simulink model "scara"  (R2023a)
settings: Solver=VariableStepAuto  StartTime=0.0  StopTime=7  MaxStep=1e-3  RelTol=1e-3
model workspace: external: MATLAB File C:\Users\Shantanu Baranwal\Desktop\simscape\scara_DataFile1.m (data not in the file)
undefined symbols (not defined in the file or in its folder): DiscIntNeverNeededParam, K, Lambda, smiData, tau, X, x0, Y, Z
libraries: sm_lib x40, nesl_utility x32, fl_lib x32, slpidlib x6, SignalEditorBlockLib x6, ee_lib x2, simulink x2, spspowerguiLib x1
(part 3 of 3)

== system scara/Subsystem4/Subsystem2/Network Coupler (Flexible Shaft) ==
  note: Uncomment rate transition
      | blocks if one or both networks
      | are running fixed step.
  note: Connect Port 1 to the network
      | with the smaller sample time, or
      | the network running variable step.
  Port 1 Interface : Subsystem  mask(Network Coupler (Flexible Shaft) Port 1 Interface){interfaceModel=an actual shaft compliance, k=0.1, lambda=0.01, samplingType=Variable step at ports 1 and 2, ts=0.001, h1=0.001, h2=0.01, predictionDiscreteToContinuous=off, smoothingContinuousToDiscrete=off, predictionSlowToFast=off, smoothingFastToSlow=off, nSmooth=1, tsSmoothing=0.01, J1=0.01, J2=0.01, tsRecommended=0.0026611, hRecommended=0.00026611, kDerived=250, lambdaDerived=20, tsMax=0.11975, through0=0}
      mask prompts: interfaceModel "physmod:simscape:couplers:SimscapeNetworkCouplersLib:SeparateUsing_MP"; k "physmod:simscape:couplers:SimscapeNetworkCouplersLib:ShaftStiffnessNmrad_MP"; lambda "physmod:simscape:couplers:SimscapeNetworkCouplersLib:ShaftDampingNmrads_MP"; samplingType "physmod:simscape:couplers:SimscapeNetworkCouplersLib:SamplingType_MP"; ts "physmod:simscape:couplers:SimscapeNetworkCouplersLib:SeparatorTimeConstants_MP"; h1 "physmod:simscape:couplers:SimscapeNetworkCouplersLib:Port1NetworkDiscreteSampleTimes_MP"; h2 "physmod:simscape:couplers:SimscapeNetworkCouplersLib:Port2NetworkDiscreteSampleTimes_MP"; predictionDiscreteToContinuous "physmod:simscape:couplers:SimscapeNetworkCouplersLib:UsePredictionWhenConnectingFixedStepToVariableStep_MP"; smoothingContinuousToDiscrete "physmod:simscape:couplers:SimscapeNetworkCouplersLib:UseSmoothingWhenConnectingVariableStepToFixedStep_MP"; predictionSlowToFast "physmod:simscape:couplers:SimscapeNetworkCouplersLib:UsePredictionWhenConnectingSlowToFastSampleTimes_MP"; smoothingFastToSlow "physmod:simscape:couplers:SimscapeNetworkCouplersLib:UseSmoothingWhenConnectingFastToSlowSampleTimes_MP"; nSmooth "physmod:simscape:couplers:SimscapeNetworkCouplersLib:NumberOfSamplesOverWhichToSmooth_MP"; tsSmoothing "physmod:simscape:couplers:SimscapeNetworkCouplersLib:SmoothingTimeConstants_MP"; J1 "physmod:simscape:couplers:SimscapeNetworkCouplersLib:ApproximateInertiaAtPort1kgm2_MP"; J2 "physmod:simscape:couplers:SimscapeNetworkCouplersLib:ApproximateInertiaAtPort2kgm2_MP"; tsRecommended "physmod:simscape:couplers:SimscapeNetworkCouplersLib:RecommendedMaxFilterTimeConstants_MP"; hRecommended "physmod:simscape:couplers:SimscapeNetworkCouplersLib:RecommendedMaxDiscreteSampleTimes_MP"; kDerived "physmod:simscape:couplers:SimscapeNetworkCouplersLib:CalculatedShaftStiffnessNmrad_MP"; lambdaDerived "physmod:simscape:couplers:SimscapeNetworkCouplersLib:CalculatedShaftDampingNmrads_MP"; tsMax "physmod:simscape:couplers:SimscapeNetworkCouplersLib:CalculatedFastestTrackableTimeConstants_MP"; through0 "physmod:simscape:couplers:SimscapeNetworkCouplersLib:InitialTransmittedTorqueNm_MP"
      mask help: physmod:simscape:couplers:SimscapeNetworkCouplersLib:NetworkCouplerFlexibleShaftPort1Interface_MD
      mask init:
      | % Fixed step sample time value check
      | foundation.internal.couplers.checkSampleTimes(gcb,h1,h2);
      | 
      | % Map mask choices to Simscape block parameters  
      | [K,Lambda,tau,~,~,x0,~] = foundation.internal.couplers.mechanical.derivedParamsRotational(...
      |     gcb,ts,h1,h2,through0,k,lambda,J1,J2);
      settings: PortSchema="{\"entries\":[{\"content\":{\"sides\":[{\"content\":{\"connectorIds\":[\"LConn1\"]},\"type\":\"ConnectorPlacement.EquallySpacedRectSide\",\"uuid\":\"a6d4a9fd-b5aa-40dc-ab7e-2b646b9b57bc\"},{\"content\":{\"connectorIds\":[\"Out1\",\"In1\"],\"side\":\"RIGHT\"},\"type\":\"ConnectorPlacement.EquallySpacedRectSide\",\"uuid\":\"31bb6273-5b9b-48d0-a1a2-6fbacb979b97\"},{\"content\":{\"connectorIds\":[],\"side\":\"TOP\"},\"type\":\"ConnectorPlacement.EquallySpacedRectSide\",\"uuid\":\"0f7afab2-4481-486c-9ad0-2b42c5b091a4\"}]},\"type\":\"ConnectorPlacement.EquallySpacedConnector\",\"uuid\":\"a98e47aa-cbfd-441a-b14c-c9ea515c056e\"}],\"packageUris\":[\"http://schema.mathworks.com/mf0/Connector/R2020b\"],\"version\":\"1.0\"}"
      mask Help: web([docroot '/simscape/ref/networkcouplerflexibleshaft.html'])
      mask TypeOptions interfaceModel: physmod:simscape:couplers:SimscapeNetworkCouplersLib:anActualShaftCompliance_PV | physmod:simscape:couplers:SimscapeNetworkCouplersLib:anAddedNumericalCompliance_PV
      mask Callback interfaceModel: foundation.internal.couplers.mechanical.parameterVisibilities(gcb)
      mask TypeOptions samplingType: physmod:simscape:couplers:SimscapeNetworkCouplersLib:VariableStepAtPorts1And2_PV | physmod:simscape:couplers:SimscapeNetworkCouplersLib:VariableStepAtPort1AndFixedStepAtPort2_PV | physmod:simscape:couplers:SimscapeNetworkCouplersLib:FixedStepBothPortsWithCommonSampleTime_PV | physmod:simscape:couplers:SimscapeNetworkCouplersLib:FixedStepBothPortsWithFasterSamplingAtPort1_PV
      mask Callback samplingType: foundation.internal.couplers.mechanical.parameterVisibilities(gcb)
      mask Callback predictionDiscreteToContinuous: foundation.internal.couplers.mechanical.parameterVisibilities(gcb)
      mask Callback smoothingContinuousToDiscrete: foundation.internal.couplers.mechanical.parameterVisibilities(gcb)
      mask Callback predictionSlowToFast: foundation.internal.couplers.mechanical.parameterVisibilities(gcb)
      mask Callback smoothingFastToSlow: foundation.internal.couplers.mechanical.parameterVisibilities(gcb)
      mask DialogControl Main Prompt: Main
      mask DialogControl interfaceModel Prompt: Separate using
      mask DialogControl k Prompt: Shaft stiffness (Nm/rad)
      mask DialogControl lambda Prompt: Shaft damping (Nm/(rad/s))
      mask DialogControl samplingType Prompt: Sampling type
      mask DialogControl ts Prompt: Separator time constant (s)
      mask DialogControl h1 Prompt: Port 1 network discrete sample time (s)
      mask DialogControl h2 Prompt: Port 2 network discrete sample time (s)
      mask DialogControl predictionDiscreteToContinuous Prompt: Use prediction when connecting fixed step to variable step
      mask DialogControl smoothingContinuousToDiscrete Prompt: Use smoothing when connecting variable step to fixed step
      mask DialogControl predictionSlowToFast Prompt: Use prediction when connecting slow to fast sample times
      mask DialogControl smoothingFastToSlow Prompt: Use smoothing when connecting fast to slow sample times
      mask DialogControl nSmooth Prompt: Number of samples over which to smooth
      mask DialogControl tsSmoothing Prompt: Smoothing time constant (s)
      mask DialogControl Analysis Prompt: Analysis
      mask DialogControl connectedNetworkInfo Prompt: Connected network information
      mask DialogControl J1 Prompt: Approximate inertia at port 1 (kg*m^2)
      mask DialogControl J2 Prompt: Approximate inertia at port 2 (kg*m^2)
      mask DialogControl derivedValues Prompt: Derived values
      mask DialogControl tsRecommended Prompt: Recommended max filter time constant (s)
      mask DialogControl hRecommended Prompt: Recommended max discrete sample time (s)
      mask DialogControl kDerived Prompt: Calculated shaft stiffness (Nm/rad)
      mask DialogControl lambdaDerived Prompt: Calculated shaft damping (Nm/(rad/s))
      mask DialogControl tsMax Prompt: Calculated fastest trackable time constant (s)
      mask DialogControl updateRecommendations Prompt: Update
      mask DialogControl updateRecommendations Callback: foundation.internal.couplers.mechanical.analysisRotational(gcb);
      mask DialogControl InitialConditions Prompt: Initial Conditions
      mask DialogControl through0 Prompt: Initial transmitted torque (Nm)
  Port 2 Interface : Subsystem  mask(Network Coupler (Flexible Shaft) Port 2 Interface){}
      mask help: physmod:simscape:couplers:SimscapeNetworkCouplersLib:NetworkCouplerFlexibleShaftPort2Interface_MD
      settings: PortSchema="{\"entries\":[{\"content\":{\"sides\":[{\"content\":{\"connectorIds\":[\"In1\",\"Out1\"]},\"type\":\"ConnectorPlacement.EquallySpacedRectSide\",\"uuid\":\"5a4c1550-e77d-42df-bf3e-b81963920de7\"},{\"content\":{\"connectorIds\":[\"RConn1\"],\"side\":\"RIGHT\"},\"type\":\"ConnectorPlacement.EquallySpacedRectSide\",\"uuid\":\"3fd730f7-5937-4563-a365-595aaae9027b\"},{\"content\":{\"connectorIds\":[],\"side\":\"TOP\"},\"type\":\"ConnectorPlacement.EquallySpacedRectSide\",\"uuid\":\"c16e04e4-26e8-4fd6-98d3-59adbef44c0d\"}]},\"type\":\"ConnectorPlacement.EquallySpacedConnector\",\"uuid\":\"5588d8d0-d459-45fe-a303-1ca6654e99d0\"}],\"packageUris\":[\"http://schema.mathworks.com/mf0/Connector/R2020b\"],\"version\":\"1.0\"}"
      mask Help: web([docroot '/simscape/ref/networkcouplerflexibleshaft.html'])
  Rate transition (fast-to-slow) : RateTransition  Commented=through  Integrity=off
  Rate transition (slow-to-fast) : RateTransition  Commented=through  Integrity=off
  1 : PMIOPort  Side=Left
  2 : PMIOPort  Port=2  Side=Right
  wires:
  Port 1 Interface/1(torque) -> Rate transition (fast-to-slow)/1
  Rate transition (fast-to-slow)/1 -> Port 2 Interface/1(torque)
  Port 2 Interface/1(speed) -> Rate transition (slow-to-fast)/1
  Rate transition (slow-to-fast)/1 -> Port 1 Interface/1(speed)
  connections:
  2/RConn1 -- Port 2 Interface/RConn1
  1/RConn1 -- Port 1 Interface/LConn1

== system scara/Subsystem4/Subsystem3/Network Coupler (Flexible Shaft) ==
  note: Connect Port 1 to the network
      | with the smaller sample time, or
      | the network running variable step.
  note: Uncomment rate transition
      | blocks if one or both networks
      | are running fixed step.
  Port 1 Interface : Subsystem  mask(Network Coupler (Flexible Shaft) Port 1 Interface){interfaceModel=an actual shaft compliance, k=0.1, lambda=0.01, samplingType=Variable step at ports 1 and 2, ts=0.001, h1=0.001, h2=0.01, predictionDiscreteToContinuous=off, smoothingContinuousToDiscrete=off, predictionSlowToFast=off, smoothingFastToSlow=off, nSmooth=1, tsSmoothing=0.01, J1=0.01, J2=0.01, tsRecommended=0.0026611, hRecommended=0.00026611, kDerived=250, lambdaDerived=20, tsMax=0.11975, through0=0}
      mask prompts: interfaceModel "physmod:simscape:couplers:SimscapeNetworkCouplersLib:SeparateUsing_MP"; k "physmod:simscape:couplers:SimscapeNetworkCouplersLib:ShaftStiffnessNmrad_MP"; lambda "physmod:simscape:couplers:SimscapeNetworkCouplersLib:ShaftDampingNmrads_MP"; samplingType "physmod:simscape:couplers:SimscapeNetworkCouplersLib:SamplingType_MP"; ts "physmod:simscape:couplers:SimscapeNetworkCouplersLib:SeparatorTimeConstants_MP"; h1 "physmod:simscape:couplers:SimscapeNetworkCouplersLib:Port1NetworkDiscreteSampleTimes_MP"; h2 "physmod:simscape:couplers:SimscapeNetworkCouplersLib:Port2NetworkDiscreteSampleTimes_MP"; predictionDiscreteToContinuous "physmod:simscape:couplers:SimscapeNetworkCouplersLib:UsePredictionWhenConnectingFixedStepToVariableStep_MP"; smoothingContinuousToDiscrete "physmod:simscape:couplers:SimscapeNetworkCouplersLib:UseSmoothingWhenConnectingVariableStepToFixedStep_MP"; predictionSlowToFast "physmod:simscape:couplers:SimscapeNetworkCouplersLib:UsePredictionWhenConnectingSlowToFastSampleTimes_MP"; smoothingFastToSlow "physmod:simscape:couplers:SimscapeNetworkCouplersLib:UseSmoothingWhenConnectingFastToSlowSampleTimes_MP"; nSmooth "physmod:simscape:couplers:SimscapeNetworkCouplersLib:NumberOfSamplesOverWhichToSmooth_MP"; tsSmoothing "physmod:simscape:couplers:SimscapeNetworkCouplersLib:SmoothingTimeConstants_MP"; J1 "physmod:simscape:couplers:SimscapeNetworkCouplersLib:ApproximateInertiaAtPort1kgm2_MP"; J2 "physmod:simscape:couplers:SimscapeNetworkCouplersLib:ApproximateInertiaAtPort2kgm2_MP"; tsRecommended "physmod:simscape:couplers:SimscapeNetworkCouplersLib:RecommendedMaxFilterTimeConstants_MP"; hRecommended "physmod:simscape:couplers:SimscapeNetworkCouplersLib:RecommendedMaxDiscreteSampleTimes_MP"; kDerived "physmod:simscape:couplers:SimscapeNetworkCouplersLib:CalculatedShaftStiffnessNmrad_MP"; lambdaDerived "physmod:simscape:couplers:SimscapeNetworkCouplersLib:CalculatedShaftDampingNmrads_MP"; tsMax "physmod:simscape:couplers:SimscapeNetworkCouplersLib:CalculatedFastestTrackableTimeConstants_MP"; through0 "physmod:simscape:couplers:SimscapeNetworkCouplersLib:InitialTransmittedTorqueNm_MP"
      mask help: physmod:simscape:couplers:SimscapeNetworkCouplersLib:NetworkCouplerFlexibleShaftPort1Interface_MD
      mask init: same as scara/Subsystem4/Subsystem2/Network Coupler (Flexible Shaft)/Port 1 Interface
      settings: PortSchema="{\"entries\":[{\"content\":{\"sides\":[{\"content\":{\"connectorIds\":[\"LConn1\"]},\"type\":\"ConnectorPlacement.EquallySpacedRectSide\",\"uuid\":\"a6d4a9fd-b5aa-40dc-ab7e-2b646b9b57bc\"},{\"content\":{\"connectorIds\":[\"Out1\",\"In1\"],\"side\":\"RIGHT\"},\"type\":\"ConnectorPlacement.EquallySpacedRectSide\",\"uuid\":\"31bb6273-5b9b-48d0-a1a2-6fbacb979b97\"},{\"content\":{\"connectorIds\":[],\"side\":\"TOP\"},\"type\":\"ConnectorPlacement.EquallySpacedRectSide\",\"uuid\":\"0f7afab2-4481-486c-9ad0-2b42c5b091a4\"}]},\"type\":\"ConnectorPlacement.EquallySpacedConnector\",\"uuid\":\"a98e47aa-cbfd-441a-b14c-c9ea515c056e\"}],\"packageUris\":[\"http://schema.mathworks.com/mf0/Connector/R2020b\"],\"version\":\"1.0\"}"
      mask Help: web([docroot '/simscape/ref/networkcouplerflexibleshaft.html'])
      mask TypeOptions interfaceModel: physmod:simscape:couplers:SimscapeNetworkCouplersLib:anActualShaftCompliance_PV | physmod:simscape:couplers:SimscapeNetworkCouplersLib:anAddedNumericalCompliance_PV
      mask Callback interfaceModel: foundation.internal.couplers.mechanical.parameterVisibilities(gcb)
      mask TypeOptions samplingType: physmod:simscape:couplers:SimscapeNetworkCouplersLib:VariableStepAtPorts1And2_PV | physmod:simscape:couplers:SimscapeNetworkCouplersLib:VariableStepAtPort1AndFixedStepAtPort2_PV | physmod:simscape:couplers:SimscapeNetworkCouplersLib:FixedStepBothPortsWithCommonSampleTime_PV | physmod:simscape:couplers:SimscapeNetworkCouplersLib:FixedStepBothPortsWithFasterSamplingAtPort1_PV
      mask Callback samplingType: foundation.internal.couplers.mechanical.parameterVisibilities(gcb)
      mask Callback predictionDiscreteToContinuous: foundation.internal.couplers.mechanical.parameterVisibilities(gcb)
      mask Callback smoothingContinuousToDiscrete: foundation.internal.couplers.mechanical.parameterVisibilities(gcb)
      mask Callback predictionSlowToFast: foundation.internal.couplers.mechanical.parameterVisibilities(gcb)
      mask Callback smoothingFastToSlow: foundation.internal.couplers.mechanical.parameterVisibilities(gcb)
      mask DialogControl Main Prompt: Main
      mask DialogControl interfaceModel Prompt: Separate using
      mask DialogControl k Prompt: Shaft stiffness (Nm/rad)
      mask DialogControl lambda Prompt: Shaft damping (Nm/(rad/s))
      mask DialogControl samplingType Prompt: Sampling type
      mask DialogControl ts Prompt: Separator time constant (s)
      mask DialogControl h1 Prompt: Port 1 network discrete sample time (s)
      mask DialogControl h2 Prompt: Port 2 network discrete sample time (s)
      mask DialogControl predictionDiscreteToContinuous Prompt: Use prediction when connecting fixed step to variable step
      mask DialogControl smoothingContinuousToDiscrete Prompt: Use smoothing when connecting variable step to fixed step
      mask DialogControl predictionSlowToFast Prompt: Use prediction when connecting slow to fast sample times
      mask DialogControl smoothingFastToSlow Prompt: Use smoothing when connecting fast to slow sample times
      mask DialogControl nSmooth Prompt: Number of samples over which to smooth
      mask DialogControl tsSmoothing Prompt: Smoothing time constant (s)
      mask DialogControl Analysis Prompt: Analysis
      mask DialogControl connectedNetworkInfo Prompt: Connected network information
      mask DialogControl J1 Prompt: Approximate inertia at port 1 (kg*m^2)
      mask DialogControl J2 Prompt: Approximate inertia at port 2 (kg*m^2)
      mask DialogControl derivedValues Prompt: Derived values
      mask DialogControl tsRecommended Prompt: Recommended max filter time constant (s)
      mask DialogControl hRecommended Prompt: Recommended max discrete sample time (s)
      mask DialogControl kDerived Prompt: Calculated shaft stiffness (Nm/rad)
      mask DialogControl lambdaDerived Prompt: Calculated shaft damping (Nm/(rad/s))
      mask DialogControl tsMax Prompt: Calculated fastest trackable time constant (s)
      mask DialogControl updateRecommendations Prompt: Update
      mask DialogControl updateRecommendations Callback: foundation.internal.couplers.mechanical.analysisRotational(gcb);
      mask DialogControl InitialConditions Prompt: Initial Conditions
      mask DialogControl through0 Prompt: Initial transmitted torque (Nm)
  Port 2 Interface : Subsystem  mask(Network Coupler (Flexible Shaft) Port 2 Interface){}
      mask help: physmod:simscape:couplers:SimscapeNetworkCouplersLib:NetworkCouplerFlexibleShaftPort2Interface_MD
      settings: PortSchema="{\"entries\":[{\"content\":{\"sides\":[{\"content\":{\"connectorIds\":[\"In1\",\"Out1\"]},\"type\":\"ConnectorPlacement.EquallySpacedRectSide\",\"uuid\":\"5a4c1550-e77d-42df-bf3e-b81963920de7\"},{\"content\":{\"connectorIds\":[\"RConn1\"],\"side\":\"RIGHT\"},\"type\":\"ConnectorPlacement.EquallySpacedRectSide\",\"uuid\":\"3fd730f7-5937-4563-a365-595aaae9027b\"},{\"content\":{\"connectorIds\":[],\"side\":\"TOP\"},\"type\":\"ConnectorPlacement.EquallySpacedRectSide\",\"uuid\":\"c16e04e4-26e8-4fd6-98d3-59adbef44c0d\"}]},\"type\":\"ConnectorPlacement.EquallySpacedConnector\",\"uuid\":\"5588d8d0-d459-45fe-a303-1ca6654e99d0\"}],\"packageUris\":[\"http://schema.mathworks.com/mf0/Connector/R2020b\"],\"version\":\"1.0\"}"
      mask Help: web([docroot '/simscape/ref/networkcouplerflexibleshaft.html'])
  Rate transition (fast-to-slow) : RateTransition  Commented=through  Integrity=off
  Rate transition (slow-to-fast) : RateTransition  Commented=through  Integrity=off
  1 : PMIOPort  Side=Left
  2 : PMIOPort  Port=2  Side=Right
  wires:
  Rate transition (slow-to-fast)/1 -> Port 1 Interface/1(speed)
  Port 2 Interface/1(speed) -> Rate transition (slow-to-fast)/1
  Rate transition (fast-to-slow)/1 -> Port 2 Interface/1(torque)
  Port 1 Interface/1(torque) -> Rate transition (fast-to-slow)/1
  connections:
  1/RConn1 -- Port 1 Interface/LConn1
  2/RConn1 -- Port 2 Interface/RConn1

== system scara/Subsystem4/Subsystem2/Network Coupler (Flexible Shaft)/Port 1 Interface ==
  speed : Inport
  Ideal Rotational Motion Sensor1 : fl_lib/Mechanical/Mechanical Sensors/Ideal Rotational Motion Sensor  reference=foundation.enum.MeasurementReference.difference  acceleration_port=false  velocity_port=true  position_port=true  wrap_angle=simscape.enum.onoff.off  offset=0 rad
  Interface : Subsystem  Variant=on  VariantControlMode=label  VariantControl=Variant1  LabelModeActiveChoice=Continuous
      settings: PortSchema="{\"entries\":[{\"content\":{\"sides\":[{\"content\":{\"connectorIds\":[\"In1\",\"Out2\"]},\"type\":\"ConnectorPlacement.EquallySpacedRectSide\",\"uuid\":\"aa56821c-7799-44e3-b228-553c5b43a68d\"},{\"content\":{\"connectorIds\":[\"In2\",\"Out1\"],\"side\":\"RIGHT\"},\"type\":\"ConnectorPlacement.EquallySpacedRectSide\",\"uuid\":\"8658dee5-55e2-4f33-bdec-e6600ce27fc1\"},{\"content\":{\"connectorIds\":[],\"side\":\"TOP\"},\"type\":\"ConnectorPlacement.EquallySpacedRectSide\",\"uuid\":\"2effe9c6-8e61-4f0c-a39b-329d9ffc707d\"}]},\"type\":\"ConnectorPlacement.EquallySpacedConnector\",\"uuid\":\"c8fc8444-dfc7-49a5-9550-b957635f7d8f\"}],\"packageUris\":[\"http://schema.mathworks.com/mf0/Connector/R2020b\"],\"version\":\"1.0\"}"
  Mechanical Rotational Reference2 : fl_lib/Mechanical/Rotational Elements/Mechanical Rotational Reference
  Mechanical Rotational Reference3 : fl_lib/Mechanical/Rotational Elements/Mechanical Rotational Reference
  T1 : nesl_utility/Simulink-PS Converter  PhysicalDomain=network_engine_domain  SubClassName=ps_input  LeftPortType=input  RightPortType=output  PseudoPeriodic=off  Frequencies=[]  NoiseDistribution=none  NoiseParameters=[]  Unit=N*m  AffineConversion=off  FilteringAndDerivatives=zero  SimscapeFilterOrder=1  InputFilterTimeConstant=0.001  UdotUserProvided=1
  Tau1 : fl_lib/Mechanical/Mechanical Sources/Ideal Torque Source
  w1 : nesl_utility/PS-Simulink Converter  PhysicalDomain=network_engine_domain  SubClassName=ps_output  LeftPortType=input  RightPortType=output  PseudoPeriodic=off  Frequencies=[]  VectorFormat=1-D array  Unit=rad/s  AffineConversion=off
  1 : PMIOPort  Side=Left
  torque : Outport
  wires:
  Interface/1(through2) -> torque/1
  w1/1 -> Interface/1(across1)
  Interface/2(through1) -> T1/1
  speed/1 -> Interface/2(across2)
  connections:
  T1/RConn1 -- Tau1/RConn1
  Mechanical Rotational Reference3/LConn1 -- Tau1/LConn1
  Ideal Rotational Motion Sensor1/RConn2 -- w1/LConn1
  Mechanical Rotational Reference2/LConn1 -- Ideal Rotational Motion Sensor1/RConn1
  Tau1/RConn2 -- Ideal Rotational Motion Sensor1/LConn1 -- 1/RConn1

== system scara/Subsystem4/Subsystem2/Network Coupler (Flexible Shaft)/Port 2 Interface ==
  torque : Inport
  Ideal Rotational Motion Sensor2 : fl_lib/Mechanical/Mechanical Sensors/Ideal Rotational Motion Sensor  reference=foundation.enum.MeasurementReference.difference  acceleration_port=false  velocity_port=true  position_port=true  wrap_angle=simscape.enum.onoff.off  offset=0 rad
  Mechanical Rotational Reference1 : fl_lib/Mechanical/Rotational Elements/Mechanical Rotational Reference
  Mechanical Rotational Reference4 : fl_lib/Mechanical/Rotational Elements/Mechanical Rotational Reference
  T2 : nesl_utility/Simulink-PS Converter  PhysicalDomain=network_engine_domain  SubClassName=ps_input  LeftPortType=input  RightPortType=output  PseudoPeriodic=off  Frequencies=[]  NoiseDistribution=none  NoiseParameters=[]  Unit=N*m  AffineConversion=off  FilteringAndDerivatives=zero  SimscapeFilterOrder=1  InputFilterTimeConstant=0.001  UdotUserProvided=1
  Tau2 : fl_lib/Mechanical/Mechanical Sources/Ideal Torque Source
  w2 : nesl_utility/PS-Simulink Converter  PhysicalDomain=network_engine_domain  SubClassName=ps_output  LeftPortType=input  RightPortType=output  PseudoPeriodic=off  Frequencies=[]  VectorFormat=1-D array  Unit=rad/s  AffineConversion=off
  2 : PMIOPort  Side=Right
  speed : Outport
  wires:
  w2/1 -> speed/1
  torque/1 -> T2/1
  connections:
  Mechanical Rotational Reference4/LConn1 -- Tau2/LConn1
  Tau2/RConn2 -- 2/RConn1 -- Ideal Rotational Motion Sensor2/LConn1
  Ideal Rotational Motion Sensor2/RConn2 -- w2/LConn1
  Mechanical Rotational Reference1/LConn1 -- Ideal Rotational Motion Sensor2/RConn1
  T2/RConn1 -- Tau2/RConn1

== system scara/Subsystem4/Subsystem3/Network Coupler (Flexible Shaft)/Port 1 Interface ==
  speed : Inport
  Ideal Rotational Motion Sensor1 : fl_lib/Mechanical/Mechanical Sensors/Ideal Rotational Motion Sensor  reference=foundation.enum.MeasurementReference.difference  acceleration_port=false  velocity_port=true  position_port=true  wrap_angle=simscape.enum.onoff.off  offset=0 rad
  Interface : Subsystem  Variant=on  VariantControlMode=label  VariantControl=Variant1  LabelModeActiveChoice=Continuous
      settings: PortSchema="{\"entries\":[{\"content\":{\"sides\":[{\"content\":{\"connectorIds\":[\"In1\",\"Out2\"]},\"type\":\"ConnectorPlacement.EquallySpacedRectSide\",\"uuid\":\"aa56821c-7799-44e3-b228-553c5b43a68d\"},{\"content\":{\"connectorIds\":[\"In2\",\"Out1\"],\"side\":\"RIGHT\"},\"type\":\"ConnectorPlacement.EquallySpacedRectSide\",\"uuid\":\"8658dee5-55e2-4f33-bdec-e6600ce27fc1\"},{\"content\":{\"connectorIds\":[],\"side\":\"TOP\"},\"type\":\"ConnectorPlacement.EquallySpacedRectSide\",\"uuid\":\"2effe9c6-8e61-4f0c-a39b-329d9ffc707d\"}]},\"type\":\"ConnectorPlacement.EquallySpacedConnector\",\"uuid\":\"c8fc8444-dfc7-49a5-9550-b957635f7d8f\"}],\"packageUris\":[\"http://schema.mathworks.com/mf0/Connector/R2020b\"],\"version\":\"1.0\"}"
  Mechanical Rotational Reference2 : fl_lib/Mechanical/Rotational Elements/Mechanical Rotational Reference
  Mechanical Rotational Reference3 : fl_lib/Mechanical/Rotational Elements/Mechanical Rotational Reference
  T1 : nesl_utility/Simulink-PS Converter  PhysicalDomain=network_engine_domain  SubClassName=ps_input  LeftPortType=input  RightPortType=output  PseudoPeriodic=off  Frequencies=[]  NoiseDistribution=none  NoiseParameters=[]  Unit=N*m  AffineConversion=off  FilteringAndDerivatives=zero  SimscapeFilterOrder=1  InputFilterTimeConstant=0.001  UdotUserProvided=1
  Tau1 : fl_lib/Mechanical/Mechanical Sources/Ideal Torque Source
  w1 : nesl_utility/PS-Simulink Converter  PhysicalDomain=network_engine_domain  SubClassName=ps_output  LeftPortType=input  RightPortType=output  PseudoPeriodic=off  Frequencies=[]  VectorFormat=1-D array  Unit=rad/s  AffineConversion=off
  1 : PMIOPort  Side=Left
  torque : Outport
  wires:
  speed/1 -> Interface/2(across2)
  Interface/2(through1) -> T1/1
  w1/1 -> Interface/1(across1)
  Interface/1(through2) -> torque/1
  connections:
  1/RConn1 -- Ideal Rotational Motion Sensor1/LConn1 -- Tau1/RConn2
  Mechanical Rotational Reference2/LConn1 -- Ideal Rotational Motion Sensor1/RConn1
  Ideal Rotational Motion Sensor1/RConn2 -- w1/LConn1
  Mechanical Rotational Reference3/LConn1 -- Tau1/LConn1
  T1/RConn1 -- Tau1/RConn1

== system scara/Subsystem4/Subsystem3/Network Coupler (Flexible Shaft)/Port 2 Interface ==
  torque : Inport
  Ideal Rotational Motion Sensor2 : fl_lib/Mechanical/Mechanical Sensors/Ideal Rotational Motion Sensor  reference=foundation.enum.MeasurementReference.difference  acceleration_port=false  velocity_port=true  position_port=true  wrap_angle=simscape.enum.onoff.off  offset=0 rad
  Mechanical Rotational Reference1 : fl_lib/Mechanical/Rotational Elements/Mechanical Rotational Reference
  Mechanical Rotational Reference4 : fl_lib/Mechanical/Rotational Elements/Mechanical Rotational Reference
  T2 : nesl_utility/Simulink-PS Converter  PhysicalDomain=network_engine_domain  SubClassName=ps_input  LeftPortType=input  RightPortType=output  PseudoPeriodic=off  Frequencies=[]  NoiseDistribution=none  NoiseParameters=[]  Unit=N*m  AffineConversion=off  FilteringAndDerivatives=zero  SimscapeFilterOrder=1  InputFilterTimeConstant=0.001  UdotUserProvided=1
  Tau2 : fl_lib/Mechanical/Mechanical Sources/Ideal Torque Source
  w2 : nesl_utility/PS-Simulink Converter  PhysicalDomain=network_engine_domain  SubClassName=ps_output  LeftPortType=input  RightPortType=output  PseudoPeriodic=off  Frequencies=[]  VectorFormat=1-D array  Unit=rad/s  AffineConversion=off
  2 : PMIOPort  Side=Right
  speed : Outport
  wires:
  torque/1 -> T2/1
  w2/1 -> speed/1
  connections:
  T2/RConn1 -- Tau2/RConn1
  Mechanical Rotational Reference1/LConn1 -- Ideal Rotational Motion Sensor2/RConn1
  Ideal Rotational Motion Sensor2/RConn2 -- w2/LConn1
  Ideal Rotational Motion Sensor2/LConn1 -- 2/RConn1 -- Tau2/RConn2
  Mechanical Rotational Reference4/LConn1 -- Tau2/LConn1

== system scara/Subsystem4/Subsystem2/Network Coupler (Flexible Shaft)/Port 1 Interface/Interface ==
  across1 : Inport
  across2 : Inport  Port=2
  Continuous : Subsystem  VariantControl=Continuous
  Discrete : Subsystem  VariantControl=Discrete
  through2 : Outport
  through1 : Outport  Port=2

== system scara/Subsystem4/Subsystem3/Network Coupler (Flexible Shaft)/Port 1 Interface/Interface ==
  across1 : Inport
  across2 : Inport  Port=2
  Continuous : Subsystem  VariantControl=Continuous
  Discrete : Subsystem  VariantControl=Discrete
  through2 : Outport
  through1 : Outport  Port=2

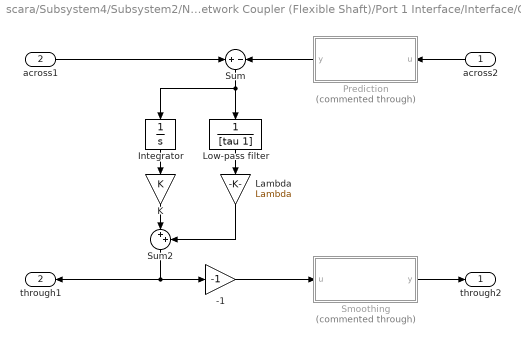
== system scara/Subsystem4/Subsystem2/Network Coupler (Flexible Shaft)/Port 1 Interface/Interface/Continuous ==
  across2 : Inport
  across1 : Inport  Port=2
  -1 : Gain  Gain=-1  SaturateOnIntegerOverflow=on  OutDataTypeStr=Inherit: Same as input  ParamDataTypeStr=Inherit: Same as input
  Integrator : Integrator  InitialCondition=x0
  K : Gain  Gain=K  SaturateOnIntegerOverflow=on  OutDataTypeStr=Inherit: Same as input  ParamDataTypeStr=Inherit: Same as input
  Lambda : Gain  Gain=Lambda  SaturateOnIntegerOverflow=on  OutDataTypeStr=Inherit: Same as input  ParamDataTypeStr=Inherit: Same as input
  Low-pass filter : TransferFcn  Numerator=1  Denominator=[tau 1]
  Prediction : Subsystem  Commented=through  mask(Prediction (discrete->continuous)){h2=h2}
      mask prompts: h2 "physmod:simscape:couplers:SimscapeNetworkCouplersLib:PortUDiscreteSampleTimes_MP"
      mask help: physmod:simscape:couplers:SimscapeNetworkCouplersLib:Predictiondiscretecontinuous_MD
      mask DialogControl h2 Prompt: Port u discrete sample time (s)
  Smoothing : Subsystem  Commented=through  mask(Smoothing (continuous->discrete)){tsSmoothing=tsSmoothing, smoothing0=-through0}
      mask prompts: tsSmoothing "physmod:simscape:couplers:SimscapeNetworkCouplersLib:SmoothingTimeConstants_MP"; smoothing0 "physmod:simscape:couplers:SimscapeNetworkCouplersLib:InitialOutput_MP"
      mask help: physmod:simscape:couplers:SimscapeNetworkCouplersLib:Smoothingcontinuousdiscrete_MD
      mask DialogControl tsSmoothing Prompt: Smoothing time constant (s)
      mask DialogControl smoothing0 Prompt: Initial output
  Sum : Sum  Inputs=+-  InputSameDT=on  SaturateOnIntegerOverflow=on  OutDataTypeStr=Inherit: Same as first input
  Sum2 : Sum  Inputs=|++
  through2 : Outport
  through1 : Outport  Port=2
  wires:
  -1/1 -> Smoothing/1(u)
  Smoothing/1(y) -> through2/1
  Prediction/1(y) -> Sum/2
  Lambda/1 -> Sum2/2
  across1/1 -> Sum/1
  Sum/1 -> Low-pass filter/1, Integrator/1
  Integrator/1 -> K/1
  Low-pass filter/1 -> Lambda/1
  across2/1 -> Prediction/1(u)
  Sum2/1 -> -1/1, through1/1
  K/1 -> Sum2/1

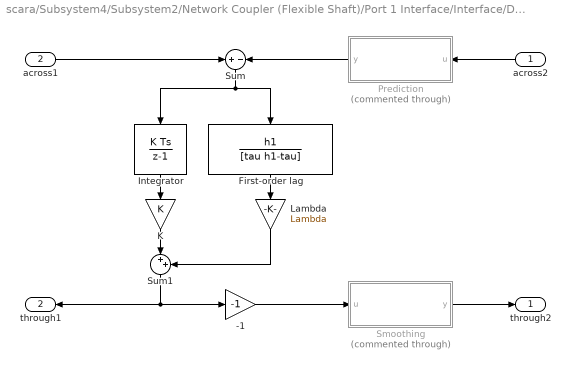
== system scara/Subsystem4/Subsystem2/Network Coupler (Flexible Shaft)/Port 1 Interface/Interface/Discrete ==
  across2 : Inport
  across1 : Inport  Port=2
  -1 : Gain  Gain=-1  SaturateOnIntegerOverflow=on  OutDataTypeStr=Inherit: Same as input  ParamDataTypeStr=Inherit: Same as input
  First-order lag : DiscreteTransferFcn  Numerator=h1  Denominator=[tau h1-tau]  SampleTime=h1
  Integrator : DiscreteIntegrator  InitialCondition=x0  SampleTime=h1  ICPrevOutput=DiscIntNeverNeededParam  ICPrevScaledInput=DiscIntNeverNeededParam
  K : Gain  Gain=K  SaturateOnIntegerOverflow=on  OutDataTypeStr=Inherit: Same as input  ParamDataTypeStr=Inherit: Same as input
  Lambda : Gain  Gain=Lambda  SaturateOnIntegerOverflow=on  OutDataTypeStr=Inherit: Same as input  ParamDataTypeStr=Inherit: Same as input
  Prediction : Subsystem  Commented=through  mask(Prediction (slow->fast)){h2=h2, h1=h1}
      mask prompts: h2 "physmod:simscape:couplers:SimscapeNetworkCouplersLib:PortUDiscreteSampleTimes_MP"; h1 "physmod:simscape:couplers:SimscapeNetworkCouplersLib:PortYDiscreteSampleTimes_MP"
      mask help: physmod:simscape:couplers:SimscapeNetworkCouplersLib:Predictionslowfast_MD
      mask DialogControl h2 Prompt: Port u discrete sample time (s)
      mask DialogControl h1 Prompt: Port y discrete sample time (s)
  Smoothing : Subsystem  Commented=through  mask(Smoothing (fast->slow)){nSmooth=nSmooth, h1=h1, smoothing0=-through0}
      mask prompts: nSmooth "physmod:simscape:couplers:SimscapeNetworkCouplersLib:NumberOfSamplesOverWhichToSmooth_MP"; h1 "physmod:simscape:couplers:SimscapeNetworkCouplersLib:PortUDiscreteSampleTimes_MP"; smoothing0 "physmod:simscape:couplers:SimscapeNetworkCouplersLib:InitialOutput_MP"
      mask help: physmod:simscape:couplers:SimscapeNetworkCouplersLib:Smoothingfastslow_MD
      mask DialogControl nSmooth Prompt: Number of samples over which to smooth
      mask DialogControl h1 Prompt: Port u discrete sample time (s)
      mask DialogControl smoothing0 Prompt: Initial output
  Sum : Sum  Inputs=+-  InputSameDT=on  SaturateOnIntegerOverflow=on  OutDataTypeStr=Inherit: Same as first input
  Sum1 : Sum  Inputs=|++
  through2 : Outport
  through1 : Outport  Port=2
  wires:
  -1/1 -> Smoothing/1(u)
  Smoothing/1(y) -> through2/1
  Prediction/1(y) -> Sum/2
  Lambda/1 -> Sum1/2
  Sum1/1 -> -1/1, through1/1
  across2/1 -> Prediction/1(u)
  Sum/1 -> First-order lag/1, Integrator/1
  across1/1 -> Sum/1
  K/1 -> Sum1/1
  Integrator/1 -> K/1
  First-order lag/1 -> Lambda/1

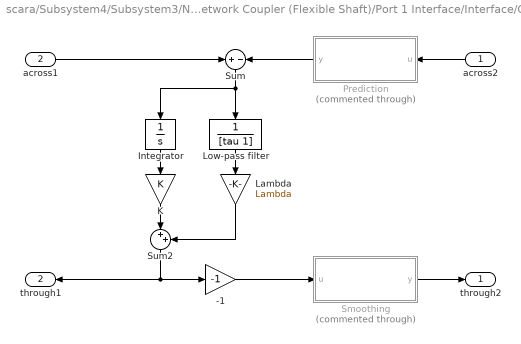
== system scara/Subsystem4/Subsystem3/Network Coupler (Flexible Shaft)/Port 1 Interface/Interface/Continuous ==
  across2 : Inport
  across1 : Inport  Port=2
  -1 : Gain  Gain=-1  SaturateOnIntegerOverflow=on  OutDataTypeStr=Inherit: Same as input  ParamDataTypeStr=Inherit: Same as input
  Integrator : Integrator  InitialCondition=x0
  K : Gain  Gain=K  SaturateOnIntegerOverflow=on  OutDataTypeStr=Inherit: Same as input  ParamDataTypeStr=Inherit: Same as input
  Lambda : Gain  Gain=Lambda  SaturateOnIntegerOverflow=on  OutDataTypeStr=Inherit: Same as input  ParamDataTypeStr=Inherit: Same as input
  Low-pass filter : TransferFcn  Numerator=1  Denominator=[tau 1]
  Prediction : Subsystem  Commented=through  mask(Prediction (discrete->continuous)){h2=h2}
      mask prompts: h2 "physmod:simscape:couplers:SimscapeNetworkCouplersLib:PortUDiscreteSampleTimes_MP"
      mask help: physmod:simscape:couplers:SimscapeNetworkCouplersLib:Predictiondiscretecontinuous_MD
      mask DialogControl h2 Prompt: Port u discrete sample time (s)
  Smoothing : Subsystem  Commented=through  mask(Smoothing (continuous->discrete)){tsSmoothing=tsSmoothing, smoothing0=-through0}
      mask prompts: tsSmoothing "physmod:simscape:couplers:SimscapeNetworkCouplersLib:SmoothingTimeConstants_MP"; smoothing0 "physmod:simscape:couplers:SimscapeNetworkCouplersLib:InitialOutput_MP"
      mask help: physmod:simscape:couplers:SimscapeNetworkCouplersLib:Smoothingcontinuousdiscrete_MD
      mask DialogControl tsSmoothing Prompt: Smoothing time constant (s)
      mask DialogControl smoothing0 Prompt: Initial output
  Sum : Sum  Inputs=+-  InputSameDT=on  SaturateOnIntegerOverflow=on  OutDataTypeStr=Inherit: Same as first input
  Sum2 : Sum  Inputs=|++
  through2 : Outport
  through1 : Outport  Port=2
  wires:
  K/1 -> Sum2/1
  Sum2/1 -> through1/1, -1/1
  across2/1 -> Prediction/1(u)
  Low-pass filter/1 -> Lambda/1
  Integrator/1 -> K/1
  Sum/1 -> Integrator/1, Low-pass filter/1
  across1/1 -> Sum/1
  Lambda/1 -> Sum2/2
  Prediction/1(y) -> Sum/2
  Smoothing/1(y) -> through2/1
  -1/1 -> Smoothing/1(u)

== system scara/Subsystem4/Subsystem3/Network Coupler (Flexible Shaft)/Port 1 Interface/Interface/Discrete ==
  across2 : Inport
  across1 : Inport  Port=2
  -1 : Gain  Gain=-1  SaturateOnIntegerOverflow=on  OutDataTypeStr=Inherit: Same as input  ParamDataTypeStr=Inherit: Same as input
  First-order lag : DiscreteTransferFcn  Numerator=h1  Denominator=[tau h1-tau]  SampleTime=h1
  Integrator : DiscreteIntegrator  InitialCondition=x0  SampleTime=h1  ICPrevOutput=DiscIntNeverNeededParam  ICPrevScaledInput=DiscIntNeverNeededParam
  K : Gain  Gain=K  SaturateOnIntegerOverflow=on  OutDataTypeStr=Inherit: Same as input  ParamDataTypeStr=Inherit: Same as input
  Lambda : Gain  Gain=Lambda  SaturateOnIntegerOverflow=on  OutDataTypeStr=Inherit: Same as input  ParamDataTypeStr=Inherit: Same as input
  Prediction : Subsystem  Commented=through  mask(Prediction (slow->fast)){h2=h2, h1=h1}
      mask prompts: h2 "physmod:simscape:couplers:SimscapeNetworkCouplersLib:PortUDiscreteSampleTimes_MP"; h1 "physmod:simscape:couplers:SimscapeNetworkCouplersLib:PortYDiscreteSampleTimes_MP"
      mask help: physmod:simscape:couplers:SimscapeNetworkCouplersLib:Predictionslowfast_MD
      mask DialogControl h2 Prompt: Port u discrete sample time (s)
      mask DialogControl h1 Prompt: Port y discrete sample time (s)
  Smoothing : Subsystem  Commented=through  mask(Smoothing (fast->slow)){nSmooth=nSmooth, h1=h1, smoothing0=-through0}
      mask prompts: nSmooth "physmod:simscape:couplers:SimscapeNetworkCouplersLib:NumberOfSamplesOverWhichToSmooth_MP"; h1 "physmod:simscape:couplers:SimscapeNetworkCouplersLib:PortUDiscreteSampleTimes_MP"; smoothing0 "physmod:simscape:couplers:SimscapeNetworkCouplersLib:InitialOutput_MP"
      mask help: physmod:simscape:couplers:SimscapeNetworkCouplersLib:Smoothingfastslow_MD
      mask DialogControl nSmooth Prompt: Number of samples over which to smooth
      mask DialogControl h1 Prompt: Port u discrete sample time (s)
      mask DialogControl smoothing0 Prompt: Initial output
  Sum : Sum  Inputs=+-  InputSameDT=on  SaturateOnIntegerOverflow=on  OutDataTypeStr=Inherit: Same as first input
  Sum1 : Sum  Inputs=|++
  through2 : Outport
  through1 : Outport  Port=2
  wires:
  First-order lag/1 -> Lambda/1
  Integrator/1 -> K/1
  K/1 -> Sum1/1
  across1/1 -> Sum/1
  Sum/1 -> Integrator/1, First-order lag/1
  across2/1 -> Prediction/1(u)
  Sum1/1 -> through1/1, -1/1
  Lambda/1 -> Sum1/2
  Prediction/1(y) -> Sum/2
  Smoothing/1(y) -> through2/1
  -1/1 -> Smoothing/1(u)

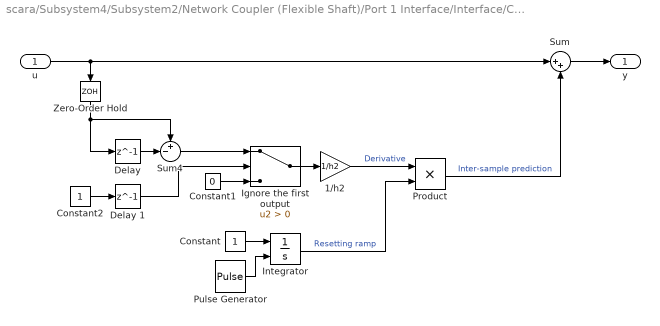
== system scara/Subsystem4/Subsystem2/Network Coupler (Flexible Shaft)/Port 1 Interface/Interface/Continuous/Prediction ==
  u : Inport
  1/h2 : Gain  Gain=1/h2
  Constant : Constant  SampleTime=h2
  Constant1 : Constant  Value=0  SampleTime=h2
  Constant2 : Constant  SampleTime=h2
  "Delay " : Delay  DelayLength=1  SampleTime=h2
  Delay 1 : Delay  DelayLength=1  SampleTime=h2
  Ignore the first output : Switch  Criteria=u2 > Threshold  SaturateOnIntegerOverflow=off  InputSameDT=off
  Integrator : Integrator  ExternalReset=either  LimitOutput=on  UpperSaturationLimit=1  LowerSaturationLimit=0
  Product : Product
  Pulse Generator : DiscretePulseGenerator  SampleTime=h2
  Sum : Sum  Inputs=|++
  Sum4 : Sum  Inputs=+-|
  Zero-Order Hold : ZeroOrderHold  SampleTime=h2
  y : Outport
  wires:
  Constant2/1 -> Delay 1/1
  Delay 1/1 -> Ignore the first output/2
  Constant1/1 -> Ignore the first output/3
  Sum4/1 -> Ignore the first output/1
  Ignore the first output/1 -> 1/h2/1
  Pulse Generator/1 -> Integrator/2
  Constant/1 -> Integrator/1
  Integrator/1 -> Product/2  "Resetting ramp"
  Sum/1 -> y/1
  1/h2/1 -> Product/1  "Derivative"
  "Delay "/1 -> Sum4/2
  u/1 -> Zero-Order Hold/1, Sum/1
  Zero-Order Hold/1 -> "Delay "/1, Sum4/1
  Product/1 -> Sum/2  "Inter-sample prediction"

== system scara/Subsystem4/Subsystem2/Network Coupler (Flexible Shaft)/Port 1 Interface/Interface/Continuous/Smoothing ==
  u : Inport
  Gain : Gain  Gain=1/tsSmoothing
  Integrator : Integrator  InitialCondition=smoothing0
  Sum : Sum  Inputs=|+-
  y : Outport
  wires:
  Sum/1 -> Gain/1
  Gain/1 -> Integrator/1
  Integrator/1 -> y/1, Sum/2
  u/1 -> Sum/1

== system scara/Subsystem4/Subsystem2/Network Coupler (Flexible Shaft)/Port 1 Interface/Interface/Discrete/Prediction ==
  u : Inport
  Constant : Constant  Value=0  SampleTime=h1
  Constant2 : Constant  Value=h1  SampleTime=h1
  "Delay " : Delay  DelayLength=1  SampleTime=h1
  Product : Product
  Resettable Delay : Delay  DelayLength=1  InitialConditionSource=Input port  ExternalReset=Rising  SampleTime=h1
      settings: InputPortMap=u0,r5,p4
  Sum : Sum  Inputs=|++
  Sum1 : Sum  Inputs=|++
  Sum4 : Sum  Inputs=+-|
  Update derivative estimate : Subsystem  TreatAsAtomicUnit=on
  y : Outport
  wires:
  Update derivative estimate/1(Out1) -> Product/1
  u/1 -> Sum/1, Sum4/1, Update derivative estimate/1(u), "Delay "/1
  "Delay "/1 -> Sum4/2
  Sum4/1 -> Update derivative estimate/Trigger, Resettable Delay/2  "Trigger when input changes"
  Sum1/1 -> Resettable Delay/1
  Resettable Delay/1 -> Product/2, Sum1/2
  Constant2/1 -> Sum1/1
  Constant/1 -> Resettable Delay/3
  Sum/1 -> y/1
  Product/1 -> Sum/2

== system scara/Subsystem4/Subsystem2/Network Coupler (Flexible Shaft)/Port 1 Interface/Interface/Discrete/Smoothing ==
  u : Inport
  Gain : Gain  Gain=1/nSmooth
  Sum of Elements : Sum  Inputs=+
  Tapped Delay : simulink/Discrete/Tapped Delay  vinit=smoothing0  samptime=h1  NumDelays=nSmooth  DelayOrder=Oldest  includeCurrent=off
  y : Outport
  wires:
  u/1 -> Tapped Delay/1
  Tapped Delay/1 -> Sum of Elements/1
  Sum of Elements/1 -> Gain/1
  Gain/1 -> y/1

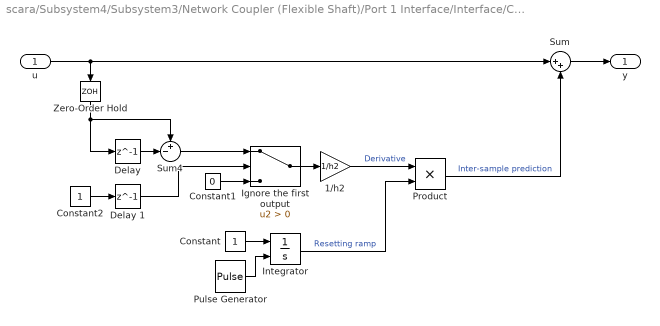
== system scara/Subsystem4/Subsystem3/Network Coupler (Flexible Shaft)/Port 1 Interface/Interface/Continuous/Prediction ==
  u : Inport
  1/h2 : Gain  Gain=1/h2
  Constant : Constant  SampleTime=h2
  Constant1 : Constant  Value=0  SampleTime=h2
  Constant2 : Constant  SampleTime=h2
  "Delay " : Delay  DelayLength=1  SampleTime=h2
  Delay 1 : Delay  DelayLength=1  SampleTime=h2
  Ignore the first output : Switch  Criteria=u2 > Threshold  SaturateOnIntegerOverflow=off  InputSameDT=off
  Integrator : Integrator  ExternalReset=either  LimitOutput=on  UpperSaturationLimit=1  LowerSaturationLimit=0
  Product : Product
  Pulse Generator : DiscretePulseGenerator  SampleTime=h2
  Sum : Sum  Inputs=|++
  Sum4 : Sum  Inputs=+-|
  Zero-Order Hold : ZeroOrderHold  SampleTime=h2
  y : Outport
  wires:
  Product/1 -> Sum/2  "Inter-sample prediction"
  Zero-Order Hold/1 -> Sum4/1, "Delay "/1
  u/1 -> Sum/1, Zero-Order Hold/1
  "Delay "/1 -> Sum4/2
  1/h2/1 -> Product/1  "Derivative"
  Sum/1 -> y/1
  Integrator/1 -> Product/2  "Resetting ramp"
  Constant/1 -> Integrator/1
  Pulse Generator/1 -> Integrator/2
  Ignore the first output/1 -> 1/h2/1
  Sum4/1 -> Ignore the first output/1
  Constant1/1 -> Ignore the first output/3
  Delay 1/1 -> Ignore the first output/2
  Constant2/1 -> Delay 1/1

== system scara/Subsystem4/Subsystem3/Network Coupler (Flexible Shaft)/Port 1 Interface/Interface/Continuous/Smoothing ==
  u : Inport
  Gain : Gain  Gain=1/tsSmoothing
  Integrator : Integrator  InitialCondition=smoothing0
  Sum : Sum  Inputs=|+-
  y : Outport
  wires:
  u/1 -> Sum/1
  Integrator/1 -> Sum/2, y/1
  Gain/1 -> Integrator/1
  Sum/1 -> Gain/1

== system scara/Subsystem4/Subsystem3/Network Coupler (Flexible Shaft)/Port 1 Interface/Interface/Discrete/Prediction ==
  u : Inport
  Constant : Constant  Value=0  SampleTime=h1
  Constant2 : Constant  Value=h1  SampleTime=h1
  "Delay " : Delay  DelayLength=1  SampleTime=h1
  Product : Product
  Resettable Delay : Delay  DelayLength=1  InitialConditionSource=Input port  ExternalReset=Rising  SampleTime=h1
      settings: InputPortMap=u0,r5,p4
  Sum : Sum  Inputs=|++
  Sum1 : Sum  Inputs=|++
  Sum4 : Sum  Inputs=+-|
  Update derivative estimate : Subsystem  TreatAsAtomicUnit=on
  y : Outport
  wires:
  Product/1 -> Sum/2
  Sum/1 -> y/1
  Constant/1 -> Resettable Delay/3
  Constant2/1 -> Sum1/1
  Resettable Delay/1 -> Sum1/2, Product/2
  Sum1/1 -> Resettable Delay/1
  Sum4/1 -> Resettable Delay/2, Update derivative estimate/Trigger  "Trigger when input changes"
  "Delay "/1 -> Sum4/2
  u/1 -> "Delay "/1, Update derivative estimate/1(u), Sum4/1, Sum/1
  Update derivative estimate/1(Out1) -> Product/1

== system scara/Subsystem4/Subsystem3/Network Coupler (Flexible Shaft)/Port 1 Interface/Interface/Discrete/Smoothing ==
  u : Inport
  Gain : Gain  Gain=1/nSmooth
  Sum of Elements : Sum  Inputs=+
  Tapped Delay : simulink/Discrete/Tapped Delay  vinit=smoothing0  samptime=h1  NumDelays=nSmooth  DelayOrder=Oldest  includeCurrent=off
  y : Outport
  wires:
  Gain/1 -> y/1
  Sum of Elements/1 -> Gain/1
  Tapped Delay/1 -> Sum of Elements/1
  u/1 -> Tapped Delay/1

== system scara/Subsystem4/Subsystem2/Network Coupler (Flexible Shaft)/Port 1 Interface/Interface/Discrete/Prediction/Update derivative estimate ==
  u : Inport
  Trigger : TriggerPort  VariantControl=(inherit)
  1/h2 : Gain  Gain=1/h2
  Constant : Constant  Value=0  SampleTime=-1
  Constant1 : Constant  SampleTime=-1
  Sum : Sum  Inputs=|-+
  Switch : Switch  Criteria=u2 > Threshold  SaturateOnIntegerOverflow=off  InputSameDT=off
  Unit Delay : UnitDelay  SampleTime=-1  HasFrameUpgradeWarning=on
  Wait one sample : UnitDelay  SampleTime=-1  HasFrameUpgradeWarning=on
  Out1 : Outport
  wires:
  Constant1/1 -> Wait one sample/1
  Wait one sample/1 -> Switch/2
  Constant/1 -> Switch/3
  Sum/1 -> Switch/1
  Switch/1 -> 1/h2/1
  1/h2/1 -> Out1/1
  u/1 -> Sum/2, Unit Delay/1
  Unit Delay/1 -> Sum/1

== system scara/Subsystem4/Subsystem3/Network Coupler (Flexible Shaft)/Port 1 Interface/Interface/Discrete/Prediction/Update derivative estimate ==
  u : Inport
  Trigger : TriggerPort  VariantControl=(inherit)
  1/h2 : Gain  Gain=1/h2
  Constant : Constant  Value=0  SampleTime=-1
  Constant1 : Constant  SampleTime=-1
  Sum : Sum  Inputs=|-+
  Switch : Switch  Criteria=u2 > Threshold  SaturateOnIntegerOverflow=off  InputSameDT=off
  Unit Delay : UnitDelay  SampleTime=-1  HasFrameUpgradeWarning=on
  Wait one sample : UnitDelay  SampleTime=-1  HasFrameUpgradeWarning=on
  Out1 : Outport
  wires:
  Unit Delay/1 -> Sum/1
  u/1 -> Unit Delay/1, Sum/2
  1/h2/1 -> Out1/1
  Switch/1 -> 1/h2/1
  Sum/1 -> Switch/1
  Constant/1 -> Switch/3
  Wait one sample/1 -> Switch/2
  Constant1/1 -> Wait one sample/1

== matlab function scara/MATLAB Function2 ==
  data: X input; theta1 output; Y input; Z input; theta2 output; d output
function [theta1,theta2,d] = IK(X,Y,Z)

l1 = 250; % length of first arm
l2 = 250; % length of second arm
if(Z<-140)
    Z = -100;
end
c2 = (X.^2 + Y.^2 - l1^2 - l2^2)/(2*l1*l2);
s2 = sqrt(1 - c2.^2);
theta2 = atan2(s2,c2);
theta1 = atan2(Y,X)-atan2(l2*sin(theta2),l1+l2*cos(theta2));
d = Z ;
%data1 = [X(:) Y(:) THETA1(:)]; % create x-y-theta1 dataset
%data2 = [X(:) Y(:) THETA2(:)]; % create x-y-theta2 dataset

== matlab function scara/MATLAB Function3 ==
  data: theta1 input; Xa output; theta2 input; d input; Ya output; z output
function [Xa,Ya,z] = FK(theta1,theta2,d)

l1 = 250;
l2 = 250;

Xa = l1*cos(theta1) + l2*cos(theta2 + theta1);
Ya = l1*sin(theta1) + l2*sin(theta2 + theta1);
z = d;

== matlab function scara/MATLAB Function4 ==
  data: theta1 input; Xa output; theta2 input; d input; Ya output; z output
function [Xa,Ya,z] = FK(theta1,theta2,d)

l1 = 250;
l2 = 250;

Xa = l1*cos(theta1) + l2*cos(theta2 + theta1);
Ya = l1*sin(theta1) + l2*sin(theta2 + theta1);
z = d;

== matlab function scara/Subsystem5/MATLAB Function5 ==
  data: X input; theta1 output; Y input; Z input; theta2 output; d output
function [theta1,theta2,d] = IK(X,Y,Z)

l1 = 250; % length of first arm
l2 = 250; % length of second arm
if(Z<-140)
    Z = -100;
end
c2 = (X.^2 + Y.^2 - l1^2 - l2^2)/(2*l1*l2);
s2 = sqrt(1 - c2.^2);
theta2 = atan2(s2,c2);
theta1 = atan2(Y,X)-atan2(l2*sin(theta2),l1+l2*cos(theta2));
d = Z ;
%data1 = [X(:) Y(:) THETA1(:)]; % create x-y-theta1 dataset
%data2 = [X(:) Y(:) THETA2(:)]; % create x-y-theta2 dataset
